simulink model "Stirred_tank_heater_FLC_Xilinx"  (R2017b)
settings: Solver=VariableStepAuto  StartTime=0.0  StopTime=4  RelTol=1e-3
libraries: xbsIndex_r4 x251
(part 2 of 2)

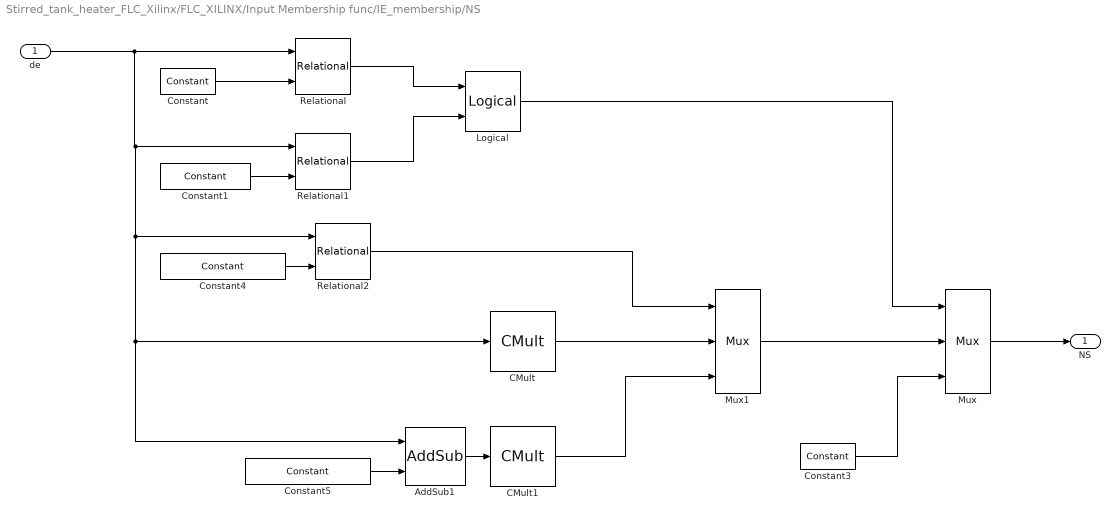
== system Stirred_tank_heater_FLC_Xilinx/FLC_XILINX/Input Membership func/IE_membership/NS ==
  de : Inport
  AddSub1 : xbsIndex_r4/AddSub  mode=Addition  use_carryin=off  use_carryout=off  en=off  latency=1  precision=Full  arith_type=Unsigned  n_bits=16  bin_pt=14  quantization=Truncate  overflow=Wrap  use_behavioral_HDL=off  hw_selection=Fabric  pipelined=off  dbl_ovrd=off  block_type=addsub
  CMult : xbsIndex_r4/CMult  const=-1/5  gui_display_data_type=Floating-point  const_n_bits=16  const_bin_pt=14  float_type=Double  exp_bits=8  fraction_bits=24  en=off  latency=1  precision=Full  arith_type="Signed  (2's comp)"  n_bits=16  bin_pt=14  quantization=Truncate  overflow=Wrap  use_behavioral_HDL=off  mem_type=Distributed RAM  pipeline=off  dbl_ovrd=off  block_type=cmult
  CMult1 : xbsIndex_r4/CMult  const=1/5  gui_display_data_type=Floating-point  const_n_bits=16  const_bin_pt=14  float_type=Double  exp_bits=8  fraction_bits=24  en=off  latency=1  precision=Full  arith_type="Signed  (2's comp)"  n_bits=16  bin_pt=14  quantization=Truncate  overflow=Wrap  use_behavioral_HDL=off  mem_type=Distributed RAM  pipeline=off  dbl_ovrd=off  block_type=cmult
  Constant : xbsIndex_r4/Constant  const=-10  gui_display_data_type=Floating-point  arith_type=Floating-point  n_bits=16  bin_pt=14  preci_type=Double  exp_width=8  frac_width=24  explicit_period=off  period=1  equ=P=C  opselect=C  inp2=PCIN>>17  opr=+  inp1=P  carry=CIN  dbl_ovrd=off  block_type=constant
  Constant1 : xbsIndex_r4/Constant  const=0  gui_display_data_type=Floating-point  arith_type=Floating-point  n_bits=16  bin_pt=14  preci_type=Double  exp_width=8  frac_width=24  explicit_period=off  period=1  equ=P=C  opselect=C  inp2=PCIN>>17  opr=+  inp1=P  carry=CIN  dbl_ovrd=off  block_type=constant
  Constant3 : xbsIndex_r4/Constant  const=0  gui_display_data_type=Floating-point  arith_type=Floating-point  n_bits=16  bin_pt=14  preci_type=Double  exp_width=8  frac_width=24  explicit_period=off  period=1  equ=P=C  opselect=C  inp2=PCIN>>17  opr=+  inp1=P  carry=CIN  dbl_ovrd=off  block_type=constant
  Constant4 : xbsIndex_r4/Constant  const=-5  gui_display_data_type=Floating-point  arith_type=Floating-point  n_bits=16  bin_pt=14  preci_type=Double  exp_width=8  frac_width=24  explicit_period=off  period=1  equ=P=C  opselect=C  inp2=PCIN>>17  opr=+  inp1=P  carry=CIN  dbl_ovrd=off  block_type=constant
  Constant5 : xbsIndex_r4/Constant  const=10  gui_display_data_type=Floating-point  arith_type=Floating-point  n_bits=16  bin_pt=14  preci_type=Double  exp_width=8  frac_width=24  explicit_period=off  period=1  equ=P=C  opselect=C  inp2=PCIN>>17  opr=+  inp1=P  carry=CIN  dbl_ovrd=off  block_type=constant
  Logical : xbsIndex_r4/Logical  logical_function=OR  inputs=2  en=off  latency=1  precision=Full  arith_type=Unsigned  n_bits=16  bin_pt=0  align_bp=on  dbl_ovrd=off  block_type=logical
  Mux : xbsIndex_r4/Mux  inputs=2  en=off  latency=1  precision=Full  arith_type=Unsigned  n_bits=16  bin_pt=14  quantization=Truncate  overflow=Wrap  dbl_ovrd=off  block_type=mux
  Mux1 : xbsIndex_r4/Mux  inputs=2  en=off  latency=1  precision=Full  arith_type=Unsigned  n_bits=16  bin_pt=14  quantization=Truncate  overflow=Wrap  dbl_ovrd=off  block_type=mux
  Relational : xbsIndex_r4/Relational  mode=a<b  op_type=Bool  en=off  latency=1  dbl_ovrd=off  block_type=relational
  Relational1 : xbsIndex_r4/Relational  mode=a>b  op_type=Bool  en=off  latency=1  dbl_ovrd=off  block_type=relational
  Relational2 : xbsIndex_r4/Relational  mode=a<b  op_type=Bool  en=off  latency=1  dbl_ovrd=off  block_type=relational
  NS : Outport
  wires:
  Constant1/1 -> Relational1/2
  Mux/1 -> NS/1
  Logical/1 -> Mux/1
  Relational/1 -> Logical/1
  Constant/1 -> Relational/2
  Constant3/1 -> Mux/3
  Relational1/1 -> Logical/2
  de/1 -> Relational2/1, CMult/1, AddSub1/1, Relational1/1, Relational/1
  Constant4/1 -> Relational2/2
  Relational2/1 -> Mux1/1
  AddSub1/1 -> CMult1/1
  Constant5/1 -> AddSub1/2
  CMult1/1 -> Mux1/3
  CMult/1 -> Mux1/2
  Mux1/1 -> Mux/2

== system Stirred_tank_heater_FLC_Xilinx/FLC_XILINX/Input Membership func/IE_membership/PB ==
  de : Inport
  AddSub : xbsIndex_r4/AddSub  mode=Subtraction  use_carryin=off  use_carryout=off  en=off  latency=1  precision=Full  arith_type=Unsigned  n_bits=16  bin_pt=14  quantization=Truncate  overflow=Wrap  use_behavioral_HDL=off  hw_selection=Fabric  pipelined=off  dbl_ovrd=off  block_type=addsub
  CMult : xbsIndex_r4/CMult  const=1/0.675  gui_display_data_type=Floating-point  const_n_bits=16  const_bin_pt=14  float_type=Double  exp_bits=8  fraction_bits=24  en=off  latency=1  precision=Full  arith_type="Signed  (2's comp)"  n_bits=16  bin_pt=14  quantization=Truncate  overflow=Wrap  use_behavioral_HDL=off  mem_type=Distributed RAM  pipeline=off  dbl_ovrd=off  block_type=cmult
  Constant : xbsIndex_r4/Constant  const=1.825  gui_display_data_type=Floating-point  arith_type=Floating-point  n_bits=16  bin_pt=14  preci_type=Double  exp_width=8  frac_width=24  explicit_period=off  period=1  equ=P=C  opselect=C  inp2=PCIN>>17  opr=+  inp1=P  carry=CIN  dbl_ovrd=off  block_type=constant
  Constant1 : xbsIndex_r4/Constant  const=2.5  gui_display_data_type=Floating-point  arith_type=Floating-point  n_bits=16  bin_pt=14  preci_type=Double  exp_width=8  frac_width=24  explicit_period=off  period=1  equ=P=C  opselect=C  inp2=PCIN>>17  opr=+  inp1=P  carry=CIN  dbl_ovrd=off  block_type=constant
  Constant2 : xbsIndex_r4/Constant  const=1.825  gui_display_data_type=Floating-point  arith_type=Floating-point  n_bits=16  bin_pt=14  preci_type=Double  exp_width=8  frac_width=24  explicit_period=off  period=1  equ=P=C  opselect=C  inp2=PCIN>>17  opr=+  inp1=P  carry=CIN  dbl_ovrd=off  block_type=constant
  Constant3 : xbsIndex_r4/Constant  const=0  gui_display_data_type=Floating-point  arith_type=Floating-point  n_bits=16  bin_pt=14  preci_type=Double  exp_width=8  frac_width=24  explicit_period=off  period=1  equ=P=C  opselect=C  inp2=PCIN>>17  opr=+  inp1=P  carry=CIN  dbl_ovrd=off  block_type=constant
  Logical : xbsIndex_r4/Logical  logical_function=OR  inputs=2  en=off  latency=1  precision=Full  arith_type=Unsigned  n_bits=16  bin_pt=0  align_bp=on  dbl_ovrd=off  block_type=logical
  Mux : xbsIndex_r4/Mux  inputs=2  en=off  latency=1  precision=Full  arith_type=Unsigned  n_bits=16  bin_pt=14  quantization=Truncate  overflow=Wrap  dbl_ovrd=off  block_type=mux
  Relational : xbsIndex_r4/Relational  mode=a<b  op_type=Bool  en=off  latency=1  dbl_ovrd=off  block_type=relational
  Relational1 : xbsIndex_r4/Relational  mode=a>b  op_type=Bool  en=off  latency=1  dbl_ovrd=off  block_type=relational
  PB : Outport
  wires:
  CMult/1 -> Mux/2
  de/1 -> AddSub/1, Relational1/1, Relational/1
  Constant1/1 -> Relational1/2
  Mux/1 -> PB/1
  Logical/1 -> Mux/1
  Relational/1 -> Logical/1
  Constant/1 -> Relational/2
  Constant3/1 -> Mux/3
  Relational1/1 -> Logical/2
  Constant2/1 -> AddSub/2
  AddSub/1 -> CMult/1

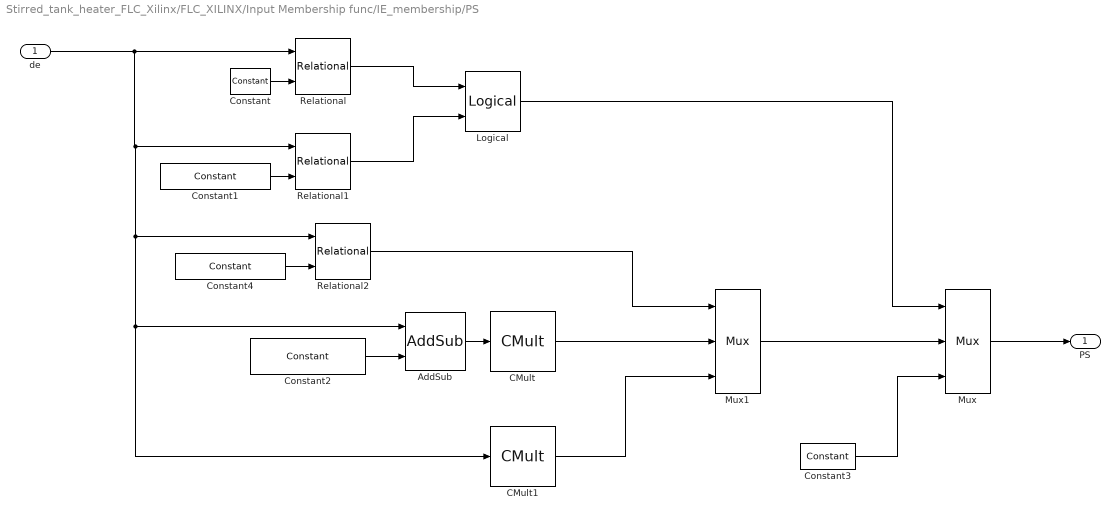
== system Stirred_tank_heater_FLC_Xilinx/FLC_XILINX/Input Membership func/IE_membership/PS ==
  de : Inport
  AddSub : xbsIndex_r4/AddSub  mode=Subtraction  use_carryin=off  use_carryout=off  en=off  latency=1  precision=Full  arith_type=Unsigned  n_bits=16  bin_pt=14  quantization=Truncate  overflow=Wrap  use_behavioral_HDL=off  hw_selection=Fabric  pipelined=off  dbl_ovrd=off  block_type=addsub
  CMult : xbsIndex_r4/CMult  const=-1/5  gui_display_data_type=Floating-point  const_n_bits=16  const_bin_pt=14  float_type=Double  exp_bits=8  fraction_bits=24  en=off  latency=1  precision=Full  arith_type="Signed  (2's comp)"  n_bits=16  bin_pt=14  quantization=Truncate  overflow=Wrap  use_behavioral_HDL=off  mem_type=Distributed RAM  pipeline=off  dbl_ovrd=off  block_type=cmult
  CMult1 : xbsIndex_r4/CMult  const=1/5  gui_display_data_type=Floating-point  const_n_bits=16  const_bin_pt=14  float_type=Double  exp_bits=8  fraction_bits=24  en=off  latency=1  precision=Full  arith_type="Signed  (2's comp)"  n_bits=16  bin_pt=14  quantization=Truncate  overflow=Wrap  use_behavioral_HDL=off  mem_type=Distributed RAM  pipeline=off  dbl_ovrd=off  block_type=cmult
  Constant : xbsIndex_r4/Constant  const=0  gui_display_data_type=Floating-point  arith_type=Floating-point  n_bits=16  bin_pt=14  preci_type=Double  exp_width=8  frac_width=24  explicit_period=off  period=1  equ=P=C  opselect=C  inp2=PCIN>>17  opr=+  inp1=P  carry=CIN  dbl_ovrd=off  block_type=constant
  Constant1 : xbsIndex_r4/Constant  const=10  gui_display_data_type=Floating-point  arith_type=Floating-point  n_bits=16  bin_pt=14  preci_type=Double  exp_width=8  frac_width=24  explicit_period=off  period=1  equ=P=C  opselect=C  inp2=PCIN>>17  opr=+  inp1=P  carry=CIN  dbl_ovrd=off  block_type=constant
  Constant2 : xbsIndex_r4/Constant  const=10  gui_display_data_type=Floating-point  arith_type=Floating-point  n_bits=16  bin_pt=14  preci_type=Double  exp_width=8  frac_width=24  explicit_period=off  period=1  equ=P=C  opselect=C  inp2=PCIN>>17  opr=+  inp1=P  carry=CIN  dbl_ovrd=off  block_type=constant
  Constant3 : xbsIndex_r4/Constant  const=0  gui_display_data_type=Floating-point  arith_type=Floating-point  n_bits=16  bin_pt=14  preci_type=Double  exp_width=8  frac_width=24  explicit_period=off  period=1  equ=P=C  opselect=C  inp2=PCIN>>17  opr=+  inp1=P  carry=CIN  dbl_ovrd=off  block_type=constant
  Constant4 : xbsIndex_r4/Constant  const=5  gui_display_data_type=Floating-point  arith_type=Floating-point  n_bits=16  bin_pt=14  preci_type=Double  exp_width=8  frac_width=24  explicit_period=off  period=1  equ=P=C  opselect=C  inp2=PCIN>>17  opr=+  inp1=P  carry=CIN  dbl_ovrd=off  block_type=constant
  Logical : xbsIndex_r4/Logical  logical_function=OR  inputs=2  en=off  latency=1  precision=Full  arith_type=Unsigned  n_bits=16  bin_pt=0  align_bp=on  dbl_ovrd=off  block_type=logical
  Mux : xbsIndex_r4/Mux  inputs=2  en=off  latency=1  precision=Full  arith_type=Unsigned  n_bits=16  bin_pt=14  quantization=Truncate  overflow=Wrap  dbl_ovrd=off  block_type=mux
  Mux1 : xbsIndex_r4/Mux  inputs=2  en=off  latency=1  precision=Full  arith_type=Unsigned  n_bits=16  bin_pt=14  quantization=Truncate  overflow=Wrap  dbl_ovrd=off  block_type=mux
  Relational : xbsIndex_r4/Relational  mode=a<b  op_type=Bool  en=off  latency=1  dbl_ovrd=off  block_type=relational
  Relational1 : xbsIndex_r4/Relational  mode=a>b  op_type=Bool  en=off  latency=1  dbl_ovrd=off  block_type=relational
  Relational2 : xbsIndex_r4/Relational  mode=a<b  op_type=Bool  en=off  latency=1  dbl_ovrd=off  block_type=relational
  PS : Outport
  wires:
  Constant1/1 -> Relational1/2
  Mux/1 -> PS/1
  Logical/1 -> Mux/1
  Relational/1 -> Logical/1
  Constant/1 -> Relational/2
  Constant3/1 -> Mux/3
  Relational1/1 -> Logical/2
  Constant2/1 -> AddSub/2
  AddSub/1 -> CMult/1
  Constant4/1 -> Relational2/2
  Relational2/1 -> Mux1/1
  de/1 -> Relational2/1, CMult1/1, AddSub/1, Relational1/1, Relational/1
  CMult1/1 -> Mux1/3
  CMult/1 -> Mux1/2
  Mux1/1 -> Mux/2

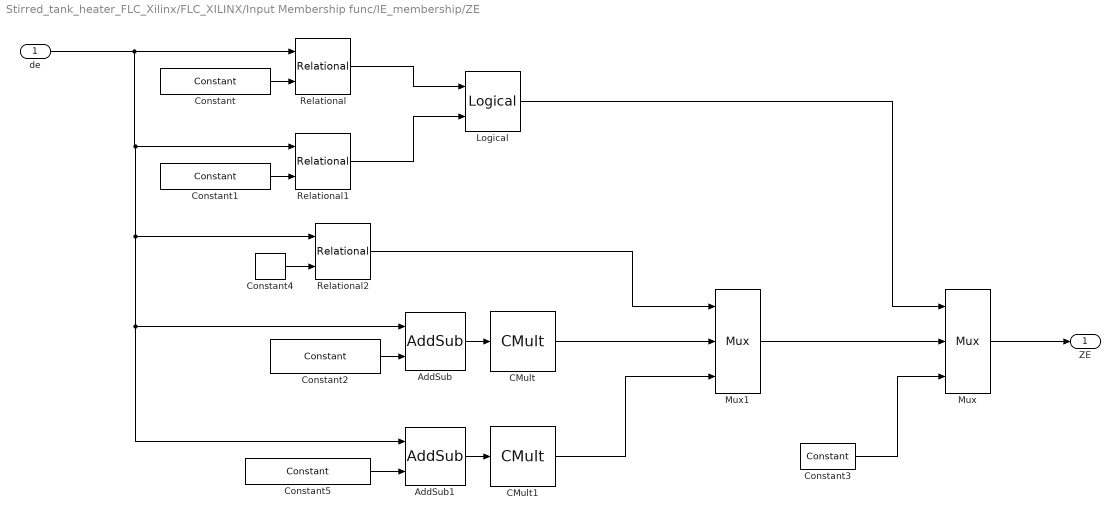
== system Stirred_tank_heater_FLC_Xilinx/FLC_XILINX/Input Membership func/IE_membership/ZE ==
  de : Inport
  AddSub : xbsIndex_r4/AddSub  mode=Subtraction  use_carryin=off  use_carryout=off  en=off  latency=1  precision=Full  arith_type=Unsigned  n_bits=16  bin_pt=14  quantization=Truncate  overflow=Wrap  use_behavioral_HDL=off  hw_selection=Fabric  pipelined=off  dbl_ovrd=off  block_type=addsub
  AddSub1 : xbsIndex_r4/AddSub  mode=Addition  use_carryin=off  use_carryout=off  en=off  latency=1  precision=Full  arith_type=Unsigned  n_bits=16  bin_pt=14  quantization=Truncate  overflow=Wrap  use_behavioral_HDL=off  hw_selection=Fabric  pipelined=off  dbl_ovrd=off  block_type=addsub
  CMult : xbsIndex_r4/CMult  const=-1/5  gui_display_data_type=Floating-point  const_n_bits=16  const_bin_pt=14  float_type=Double  exp_bits=8  fraction_bits=24  en=off  latency=1  precision=Full  arith_type="Signed  (2's comp)"  n_bits=16  bin_pt=14  quantization=Truncate  overflow=Wrap  use_behavioral_HDL=off  mem_type=Distributed RAM  pipeline=off  dbl_ovrd=off  block_type=cmult
  CMult1 : xbsIndex_r4/CMult  const=1/5  gui_display_data_type=Floating-point  const_n_bits=16  const_bin_pt=14  float_type=Double  exp_bits=8  fraction_bits=24  en=off  latency=1  precision=Full  arith_type="Signed  (2's comp)"  n_bits=16  bin_pt=14  quantization=Truncate  overflow=Wrap  use_behavioral_HDL=off  mem_type=Distributed RAM  pipeline=off  dbl_ovrd=off  block_type=cmult
  Constant : xbsIndex_r4/Constant  const=-5  gui_display_data_type=Floating-point  arith_type=Floating-point  n_bits=16  bin_pt=14  preci_type=Double  exp_width=8  frac_width=24  explicit_period=off  period=1  equ=P=C  opselect=C  inp2=PCIN>>17  opr=+  inp1=P  carry=CIN  dbl_ovrd=off  block_type=constant
  Constant1 : xbsIndex_r4/Constant  const=5  gui_display_data_type=Floating-point  arith_type=Floating-point  n_bits=16  bin_pt=14  preci_type=Double  exp_width=8  frac_width=24  explicit_period=off  period=1  equ=P=C  opselect=C  inp2=PCIN>>17  opr=+  inp1=P  carry=CIN  dbl_ovrd=off  block_type=constant
  Constant2 : xbsIndex_r4/Constant  const=5  gui_display_data_type=Floating-point  arith_type=Floating-point  n_bits=16  bin_pt=14  preci_type=Double  exp_width=8  frac_width=24  explicit_period=off  period=1  equ=P=C  opselect=C  inp2=PCIN>>17  opr=+  inp1=P  carry=CIN  dbl_ovrd=off  block_type=constant
  Constant3 : xbsIndex_r4/Constant  const=0  gui_display_data_type=Floating-point  arith_type=Floating-point  n_bits=16  bin_pt=14  preci_type=Double  exp_width=8  frac_width=24  explicit_period=off  period=1  equ=P=C  opselect=C  inp2=PCIN>>17  opr=+  inp1=P  carry=CIN  dbl_ovrd=off  block_type=constant
  Constant4 : xbsIndex_r4/Constant  const=0  gui_display_data_type=Floating-point  arith_type=Floating-point  n_bits=16  bin_pt=14  preci_type=Double  exp_width=8  frac_width=24  explicit_period=off  period=1  equ=P=C  opselect=C  inp2=PCIN>>17  opr=+  inp1=P  carry=CIN  dbl_ovrd=off  block_type=constant
  Constant5 : xbsIndex_r4/Constant  const=5  gui_display_data_type=Floating-point  arith_type=Floating-point  n_bits=16  bin_pt=14  preci_type=Double  exp_width=8  frac_width=24  explicit_period=off  period=1  equ=P=C  opselect=C  inp2=PCIN>>17  opr=+  inp1=P  carry=CIN  dbl_ovrd=off  block_type=constant
  Logical : xbsIndex_r4/Logical  logical_function=OR  inputs=2  en=off  latency=1  precision=Full  arith_type=Unsigned  n_bits=16  bin_pt=0  align_bp=on  dbl_ovrd=off  block_type=logical
  Mux : xbsIndex_r4/Mux  inputs=2  en=off  latency=1  precision=Full  arith_type=Unsigned  n_bits=16  bin_pt=14  quantization=Truncate  overflow=Wrap  dbl_ovrd=off  block_type=mux
  Mux1 : xbsIndex_r4/Mux  inputs=2  en=off  latency=1  precision=Full  arith_type=Unsigned  n_bits=16  bin_pt=14  quantization=Truncate  overflow=Wrap  dbl_ovrd=off  block_type=mux
  Relational : xbsIndex_r4/Relational  mode=a<b  op_type=Bool  en=off  latency=1  dbl_ovrd=off  block_type=relational
  Relational1 : xbsIndex_r4/Relational  mode=a>b  op_type=Bool  en=off  latency=1  dbl_ovrd=off  block_type=relational
  Relational2 : xbsIndex_r4/Relational  mode=a<b  op_type=Bool  en=off  latency=1  dbl_ovrd=off  block_type=relational
  ZE : Outport
  wires:
  Constant1/1 -> Relational1/2
  Mux/1 -> ZE/1
  Logical/1 -> Mux/1
  Relational/1 -> Logical/1
  Constant/1 -> Relational/2
  Constant3/1 -> Mux/3
  Relational1/1 -> Logical/2
  Constant2/1 -> AddSub/2
  AddSub/1 -> CMult/1
  Constant4/1 -> Relational2/2
  Relational2/1 -> Mux1/1
  AddSub1/1 -> CMult1/1
  Constant5/1 -> AddSub1/2
  de/1 -> Relational2/1, AddSub1/1, AddSub/1, Relational1/1, Relational/1
  CMult1/1 -> Mux1/3
  CMult/1 -> Mux1/2
  Mux1/1 -> Mux/2

== system Stirred_tank_heater_FLC_Xilinx/FLC_XILINX/Rules decision logic/Rules/R1 ==
  NB1 : Inport
  NB2 : Inport  Port=2
  Mux : xbsIndex_r4/Mux  inputs=2  en=off  latency=1  precision=Full  arith_type=Unsigned  n_bits=16  bin_pt=14  quantization=Truncate  overflow=Wrap  dbl_ovrd=off  block_type=mux
  Relational : xbsIndex_r4/Relational  mode=a<b  op_type=Bool  en=off  latency=1  dbl_ovrd=off  block_type=relational
  R1_NB : Outport
  wires:
  NB1/1 -> Mux/3, Relational/1
  NB2/1 -> Relational/2, Mux/2
  Mux/1 -> R1_NB/1
  Relational/1 -> Mux/1

== system Stirred_tank_heater_FLC_Xilinx/FLC_XILINX/Rules decision logic/Rules/R10 ==
  NS1 : Inport
  PB2 : Inport  Port=2
  Mux : xbsIndex_r4/Mux  inputs=2  en=off  latency=1  precision=Full  arith_type=Unsigned  n_bits=16  bin_pt=14  quantization=Truncate  overflow=Wrap  dbl_ovrd=off  block_type=mux
  Relational : xbsIndex_r4/Relational  mode=a<b  op_type=Bool  en=off  latency=1  dbl_ovrd=off  block_type=relational
  R10_PS : Outport
  wires:
  NS1/1 -> Mux/3, Relational/1
  PB2/1 -> Relational/2, Mux/2
  Mux/1 -> R10_PS/1
  Relational/1 -> Mux/1

== system Stirred_tank_heater_FLC_Xilinx/FLC_XILINX/Rules decision logic/Rules/R11 ==
  ZE1 : Inport
  NB2 : Inport  Port=2
  Mux : xbsIndex_r4/Mux  inputs=2  en=off  latency=1  precision=Full  arith_type=Unsigned  n_bits=16  bin_pt=14  quantization=Truncate  overflow=Wrap  dbl_ovrd=off  block_type=mux
  Relational : xbsIndex_r4/Relational  mode=a<b  op_type=Bool  en=off  latency=1  dbl_ovrd=off  block_type=relational
  R11_NB : Outport
  wires:
  ZE1/1 -> Mux/3, Relational/1
  NB2/1 -> Relational/2, Mux/2
  Mux/1 -> R11_NB/1
  Relational/1 -> Mux/1

== system Stirred_tank_heater_FLC_Xilinx/FLC_XILINX/Rules decision logic/Rules/R12 ==
  ZE1 : Inport
  NS2 : Inport  Port=2
  Mux : xbsIndex_r4/Mux  inputs=2  en=off  latency=1  precision=Full  arith_type=Unsigned  n_bits=16  bin_pt=14  quantization=Truncate  overflow=Wrap  dbl_ovrd=off  block_type=mux
  Relational : xbsIndex_r4/Relational  mode=a<b  op_type=Bool  en=off  latency=1  dbl_ovrd=off  block_type=relational
  R12_NS : Outport
  wires:
  ZE1/1 -> Mux/3, Relational/1
  NS2/1 -> Relational/2, Mux/2
  Mux/1 -> R12_NS/1
  Relational/1 -> Mux/1

== system Stirred_tank_heater_FLC_Xilinx/FLC_XILINX/Rules decision logic/Rules/R13 ==
  ZE1 : Inport
  ZE2 : Inport  Port=2
  Mux : xbsIndex_r4/Mux  inputs=2  en=off  latency=1  precision=Full  arith_type=Unsigned  n_bits=16  bin_pt=14  quantization=Truncate  overflow=Wrap  dbl_ovrd=off  block_type=mux
  Relational : xbsIndex_r4/Relational  mode=a<b  op_type=Bool  en=off  latency=1  dbl_ovrd=off  block_type=relational
  R13_ZE : Outport
  wires:
  ZE1/1 -> Mux/3, Relational/1
  ZE2/1 -> Relational/2, Mux/2
  Mux/1 -> R13_ZE/1
  Relational/1 -> Mux/1

== system Stirred_tank_heater_FLC_Xilinx/FLC_XILINX/Rules decision logic/Rules/R14 ==
  ZE1 : Inport
  PS2 : Inport  Port=2
  Mux : xbsIndex_r4/Mux  inputs=2  en=off  latency=1  precision=Full  arith_type=Unsigned  n_bits=16  bin_pt=14  quantization=Truncate  overflow=Wrap  dbl_ovrd=off  block_type=mux
  Relational : xbsIndex_r4/Relational  mode=a<b  op_type=Bool  en=off  latency=1  dbl_ovrd=off  block_type=relational
  R14_PS : Outport
  wires:
  ZE1/1 -> Mux/3, Relational/1
  PS2/1 -> Relational/2, Mux/2
  Mux/1 -> R14_PS/1
  Relational/1 -> Mux/1

== system Stirred_tank_heater_FLC_Xilinx/FLC_XILINX/Rules decision logic/Rules/R15 ==
  ZE1 : Inport
  PB2 : Inport  Port=2
  Mux : xbsIndex_r4/Mux  inputs=2  en=off  latency=1  precision=Full  arith_type=Unsigned  n_bits=16  bin_pt=14  quantization=Truncate  overflow=Wrap  dbl_ovrd=off  block_type=mux
  Relational : xbsIndex_r4/Relational  mode=a<b  op_type=Bool  en=off  latency=1  dbl_ovrd=off  block_type=relational
  R15_PB : Outport
  wires:
  ZE1/1 -> Mux/3, Relational/1
  PB2/1 -> Relational/2, Mux/2
  Mux/1 -> R15_PB/1
  Relational/1 -> Mux/1

== system Stirred_tank_heater_FLC_Xilinx/FLC_XILINX/Rules decision logic/Rules/R16 ==
  PS1 : Inport
  NB2 : Inport  Port=2
  Mux : xbsIndex_r4/Mux  inputs=2  en=off  latency=1  precision=Full  arith_type=Unsigned  n_bits=16  bin_pt=14  quantization=Truncate  overflow=Wrap  dbl_ovrd=off  block_type=mux
  Relational : xbsIndex_r4/Relational  mode=a<b  op_type=Bool  en=off  latency=1  dbl_ovrd=off  block_type=relational
  R16_NS : Outport
  wires:
  PS1/1 -> Mux/3, Relational/1
  NB2/1 -> Relational/2, Mux/2
  Mux/1 -> R16_NS/1
  Relational/1 -> Mux/1

== system Stirred_tank_heater_FLC_Xilinx/FLC_XILINX/Rules decision logic/Rules/R17 ==
  PS1 : Inport
  NS2 : Inport  Port=2
  Mux : xbsIndex_r4/Mux  inputs=2  en=off  latency=1  precision=Full  arith_type=Unsigned  n_bits=16  bin_pt=14  quantization=Truncate  overflow=Wrap  dbl_ovrd=off  block_type=mux
  Relational : xbsIndex_r4/Relational  mode=a<b  op_type=Bool  en=off  latency=1  dbl_ovrd=off  block_type=relational
  R17_ZE : Outport
  wires:
  PS1/1 -> Mux/3, Relational/1
  NS2/1 -> Relational/2, Mux/2
  Mux/1 -> R17_ZE/1
  Relational/1 -> Mux/1

== system Stirred_tank_heater_FLC_Xilinx/FLC_XILINX/Rules decision logic/Rules/R18 ==
  PS1 : Inport
  NE2 : Inport  Port=2
  Mux : xbsIndex_r4/Mux  inputs=2  en=off  latency=1  precision=Full  arith_type=Unsigned  n_bits=16  bin_pt=14  quantization=Truncate  overflow=Wrap  dbl_ovrd=off  block_type=mux
  Relational : xbsIndex_r4/Relational  mode=a<b  op_type=Bool  en=off  latency=1  dbl_ovrd=off  block_type=relational
  R18_PS : Outport
  wires:
  PS1/1 -> Mux/3, Relational/1
  NE2/1 -> Relational/2, Mux/2
  Mux/1 -> R18_PS/1
  Relational/1 -> Mux/1

== system Stirred_tank_heater_FLC_Xilinx/FLC_XILINX/Rules decision logic/Rules/R19 ==
  PS1 : Inport
  PS2 : Inport  Port=2
  Mux : xbsIndex_r4/Mux  inputs=2  en=off  latency=1  precision=Full  arith_type=Unsigned  n_bits=16  bin_pt=14  quantization=Truncate  overflow=Wrap  dbl_ovrd=off  block_type=mux
  Relational : xbsIndex_r4/Relational  mode=a<b  op_type=Bool  en=off  latency=1  dbl_ovrd=off  block_type=relational
  R19_PB : Outport
  wires:
  PS1/1 -> Mux/3, Relational/1
  PS2/1 -> Relational/2, Mux/2
  Mux/1 -> R19_PB/1
  Relational/1 -> Mux/1

== system Stirred_tank_heater_FLC_Xilinx/FLC_XILINX/Rules decision logic/Rules/R2 ==
  NB1 : Inport
  NS2 : Inport  Port=2
  Mux : xbsIndex_r4/Mux  inputs=2  en=off  latency=1  precision=Full  arith_type=Unsigned  n_bits=16  bin_pt=14  quantization=Truncate  overflow=Wrap  dbl_ovrd=off  block_type=mux
  Relational : xbsIndex_r4/Relational  mode=a<b  op_type=Bool  en=off  latency=1  dbl_ovrd=off  block_type=relational
  R2_NB : Outport
  wires:
  NB1/1 -> Mux/3, Relational/1
  NS2/1 -> Relational/2, Mux/2
  Mux/1 -> R2_NB/1
  Relational/1 -> Mux/1

== system Stirred_tank_heater_FLC_Xilinx/FLC_XILINX/Rules decision logic/Rules/R20 ==
  PS1 : Inport
  PB2 : Inport  Port=2
  Mux : xbsIndex_r4/Mux  inputs=2  en=off  latency=1  precision=Full  arith_type=Unsigned  n_bits=16  bin_pt=14  quantization=Truncate  overflow=Wrap  dbl_ovrd=off  block_type=mux
  Relational : xbsIndex_r4/Relational  mode=a<b  op_type=Bool  en=off  latency=1  dbl_ovrd=off  block_type=relational
  R20_PB : Outport
  wires:
  PS1/1 -> Mux/3, Relational/1
  PB2/1 -> Relational/2, Mux/2
  Mux/1 -> R20_PB/1
  Relational/1 -> Mux/1

== system Stirred_tank_heater_FLC_Xilinx/FLC_XILINX/Rules decision logic/Rules/R21 ==
  PB1 : Inport
  NB2 : Inport  Port=2
  Mux : xbsIndex_r4/Mux  inputs=2  en=off  latency=1  precision=Full  arith_type=Unsigned  n_bits=16  bin_pt=14  quantization=Truncate  overflow=Wrap  dbl_ovrd=off  block_type=mux
  Relational : xbsIndex_r4/Relational  mode=a<b  op_type=Bool  en=off  latency=1  dbl_ovrd=off  block_type=relational
  R21_ZE : Outport
  wires:
  PB1/1 -> Mux/3, Relational/1
  NB2/1 -> Relational/2, Mux/2
  Mux/1 -> R21_ZE/1
  Relational/1 -> Mux/1

== system Stirred_tank_heater_FLC_Xilinx/FLC_XILINX/Rules decision logic/Rules/R22 ==
  PB1 : Inport
  NS2 : Inport  Port=2
  Mux : xbsIndex_r4/Mux  inputs=2  en=off  latency=1  precision=Full  arith_type=Unsigned  n_bits=16  bin_pt=14  quantization=Truncate  overflow=Wrap  dbl_ovrd=off  block_type=mux
  Relational : xbsIndex_r4/Relational  mode=a<b  op_type=Bool  en=off  latency=1  dbl_ovrd=off  block_type=relational
  R22_PS : Outport
  wires:
  PB1/1 -> Mux/3, Relational/1
  NS2/1 -> Relational/2, Mux/2
  Mux/1 -> R22_PS/1
  Relational/1 -> Mux/1

== system Stirred_tank_heater_FLC_Xilinx/FLC_XILINX/Rules decision logic/Rules/R23 ==
  PB1 : Inport
  NE2 : Inport  Port=2
  Mux : xbsIndex_r4/Mux  inputs=2  en=off  latency=1  precision=Full  arith_type=Unsigned  n_bits=16  bin_pt=14  quantization=Truncate  overflow=Wrap  dbl_ovrd=off  block_type=mux
  Relational : xbsIndex_r4/Relational  mode=a<b  op_type=Bool  en=off  latency=1  dbl_ovrd=off  block_type=relational
  R23_PB : Outport
  wires:
  PB1/1 -> Mux/3, Relational/1
  NE2/1 -> Relational/2, Mux/2
  Mux/1 -> R23_PB/1
  Relational/1 -> Mux/1

== system Stirred_tank_heater_FLC_Xilinx/FLC_XILINX/Rules decision logic/Rules/R24 ==
  PB1 : Inport
  PS2 : Inport  Port=2
  Mux : xbsIndex_r4/Mux  inputs=2  en=off  latency=1  precision=Full  arith_type=Unsigned  n_bits=16  bin_pt=14  quantization=Truncate  overflow=Wrap  dbl_ovrd=off  block_type=mux
  Relational : xbsIndex_r4/Relational  mode=a<b  op_type=Bool  en=off  latency=1  dbl_ovrd=off  block_type=relational
  R24_PB : Outport
  wires:
  PB1/1 -> Mux/3, Relational/1
  PS2/1 -> Relational/2, Mux/2
  Mux/1 -> R24_PB/1
  Relational/1 -> Mux/1

== system Stirred_tank_heater_FLC_Xilinx/FLC_XILINX/Rules decision logic/Rules/R25 ==
  PB1 : Inport
  PB2 : Inport  Port=2
  Mux : xbsIndex_r4/Mux  inputs=2  en=off  latency=1  precision=Full  arith_type=Unsigned  n_bits=16  bin_pt=14  quantization=Truncate  overflow=Wrap  dbl_ovrd=off  block_type=mux
  Relational : xbsIndex_r4/Relational  mode=a<b  op_type=Bool  en=off  latency=1  dbl_ovrd=off  block_type=relational
  R25_NB : Outport
  wires:
  PB1/1 -> Mux/3, Relational/1
  PB2/1 -> Relational/2, Mux/2
  Mux/1 -> R25_NB/1
  Relational/1 -> Mux/1

== system Stirred_tank_heater_FLC_Xilinx/FLC_XILINX/Rules decision logic/Rules/R3 ==
  NB1 : Inport
  NE2 : Inport  Port=2
  Mux : xbsIndex_r4/Mux  inputs=2  en=off  latency=1  precision=Full  arith_type=Unsigned  n_bits=16  bin_pt=14  quantization=Truncate  overflow=Wrap  dbl_ovrd=off  block_type=mux
  Relational : xbsIndex_r4/Relational  mode=a<b  op_type=Bool  en=off  latency=1  dbl_ovrd=off  block_type=relational
  R3_NB : Outport
  wires:
  NB1/1 -> Mux/3, Relational/1
  NE2/1 -> Relational/2, Mux/2
  Mux/1 -> R3_NB/1
  Relational/1 -> Mux/1

== system Stirred_tank_heater_FLC_Xilinx/FLC_XILINX/Rules decision logic/Rules/R4 ==
  NB1 : Inport
  PS2 : Inport  Port=2
  Mux : xbsIndex_r4/Mux  inputs=2  en=off  latency=1  precision=Full  arith_type=Unsigned  n_bits=16  bin_pt=14  quantization=Truncate  overflow=Wrap  dbl_ovrd=off  block_type=mux
  Relational : xbsIndex_r4/Relational  mode=a<b  op_type=Bool  en=off  latency=1  dbl_ovrd=off  block_type=relational
  R4_NS : Outport
  wires:
  NB1/1 -> Mux/3, Relational/1
  PS2/1 -> Relational/2, Mux/2
  Mux/1 -> R4_NS/1
  Relational/1 -> Mux/1

== system Stirred_tank_heater_FLC_Xilinx/FLC_XILINX/Rules decision logic/Rules/R5 ==
  NB1 : Inport
  PB2 : Inport  Port=2
  Mux : xbsIndex_r4/Mux  inputs=2  en=off  latency=1  precision=Full  arith_type=Unsigned  n_bits=16  bin_pt=14  quantization=Truncate  overflow=Wrap  dbl_ovrd=off  block_type=mux
  Relational : xbsIndex_r4/Relational  mode=a<b  op_type=Bool  en=off  latency=1  dbl_ovrd=off  block_type=relational
  R5_ZE : Outport
  wires:
  NB1/1 -> Mux/3, Relational/1
  PB2/1 -> Relational/2, Mux/2
  Mux/1 -> R5_ZE/1
  Relational/1 -> Mux/1

== system Stirred_tank_heater_FLC_Xilinx/FLC_XILINX/Rules decision logic/Rules/R6 ==
  NS1 : Inport
  NB2 : Inport  Port=2
  Mux : xbsIndex_r4/Mux  inputs=2  en=off  latency=1  precision=Full  arith_type=Unsigned  n_bits=16  bin_pt=14  quantization=Truncate  overflow=Wrap  dbl_ovrd=off  block_type=mux
  Relational : xbsIndex_r4/Relational  mode=a<b  op_type=Bool  en=off  latency=1  dbl_ovrd=off  block_type=relational
  R6_NB : Outport
  wires:
  NS1/1 -> Mux/3, Relational/1
  NB2/1 -> Relational/2, Mux/2
  Mux/1 -> R6_NB/1
  Relational/1 -> Mux/1

== system Stirred_tank_heater_FLC_Xilinx/FLC_XILINX/Rules decision logic/Rules/R7 ==
  NS1 : Inport
  NS2 : Inport  Port=2
  Mux : xbsIndex_r4/Mux  inputs=2  en=off  latency=1  precision=Full  arith_type=Unsigned  n_bits=16  bin_pt=14  quantization=Truncate  overflow=Wrap  dbl_ovrd=off  block_type=mux
  Relational : xbsIndex_r4/Relational  mode=a<b  op_type=Bool  en=off  latency=1  dbl_ovrd=off  block_type=relational
  R7_NB : Outport
  wires:
  NS1/1 -> Mux/3, Relational/1
  NS2/1 -> Relational/2, Mux/2
  Mux/1 -> R7_NB/1
  Relational/1 -> Mux/1

== system Stirred_tank_heater_FLC_Xilinx/FLC_XILINX/Rules decision logic/Rules/R8 ==
  NS1 : Inport
  NE2 : Inport  Port=2
  Mux : xbsIndex_r4/Mux  inputs=2  en=off  latency=1  precision=Full  arith_type=Unsigned  n_bits=16  bin_pt=14  quantization=Truncate  overflow=Wrap  dbl_ovrd=off  block_type=mux
  Relational : xbsIndex_r4/Relational  mode=a<b  op_type=Bool  en=off  latency=1  dbl_ovrd=off  block_type=relational
  R8_NS : Outport
  wires:
  NS1/1 -> Mux/3, Relational/1
  NE2/1 -> Relational/2, Mux/2
  Mux/1 -> R8_NS/1
  Relational/1 -> Mux/1

== system Stirred_tank_heater_FLC_Xilinx/FLC_XILINX/Rules decision logic/Rules/R9 ==
  NS1 : Inport
  PS2 : Inport  Port=2
  Mux : xbsIndex_r4/Mux  inputs=2  en=off  latency=1  precision=Full  arith_type=Unsigned  n_bits=16  bin_pt=14  quantization=Truncate  overflow=Wrap  dbl_ovrd=off  block_type=mux
  Relational : xbsIndex_r4/Relational  mode=a<b  op_type=Bool  en=off  latency=1  dbl_ovrd=off  block_type=relational
  R9_ZE : Outport
  wires:
  NS1/1 -> Mux/3, Relational/1
  PS2/1 -> Relational/2, Mux/2
  Mux/1 -> R9_ZE/1
  Relational/1 -> Mux/1
